simulink model "rtwdemo_advisor2"  (Simulink 6.0)
settings: Solver=FixedStepDiscrete  SolverMode=SingleTasking  StartTime=0.0  StopTime=4  FixedStep=1  RelTol=1e-3  AbsTol=1e-6
undefined symbols (not defined in the file or in its folder): DiscIntNeverNeededParam
libraries: simulink x4, rtwdemowidgets x1
settings Model: CovMetricSettings=d  Creator=The MathWorks Inc.  LastModifiedBy=batserve  ExtModeTrigMode=oneshot  ExtModeArmWhenConnect=off  ExtModeAutoUpdateStatusClock=off  ProdHWDeviceType=Specified
settings DataIOCC: LimitDataPoints=off  SaveOutput=off  SaveTime=off  SignalLoggingName=sigsOut
settings OptimizationCC: InlineParams=on  EnforceIntegerDowncast=off  ZeroExternalMemoryAtStartup=off  ZeroInternalMemoryAtStartup=off  OptimizeModelRefInitCode=on  LifeSpan=1
settings DebuggingCC: CheckExecutionContextPreStartOutputMsg=on  CheckExecutionContextRuntimeOutputMsg=on  SolverPrmCheckMsg=none  IntegerOverflowMsg=none  ParameterDowncastMsg=warning  ParameterOverflowMsg=warning  ParameterPrecisionLossMsg=none
settings HardwareCC: ProdBitPerInt=16  ProdHWDeviceType=Specified  TargetUnknown=on
settings RTWCC: SystemTargetFile=ert.tlc  GenCodeOnly=on  TemplateMakefile=ert_default_tmf  GenerateReport=on  RTWVerbose=off  ProcessScript=ert_make_rtw_hook  IncludeHyperlinkInReport=on  LaunchReport=on
settings CodeAppCC: IgnoreCustomStorageClasses=off  IncHierarchyInIds=on  IncDataTypeInIds=on
settings ERTTargetCC: TargetFcnLib=ansi_tfl_tmw.mat  GenFloatMathFcnCalls=ANSI_C  IncludeMdlTerminateFcn=off  SuppressErrorStatus=on  SupportContinuousTime=on  SupportNonInlinedSFcns=on  RootIOFormat=Individual Arguments  ERTCustomFileTemplate=example_file_process.tlc  InitialValueSource=Model

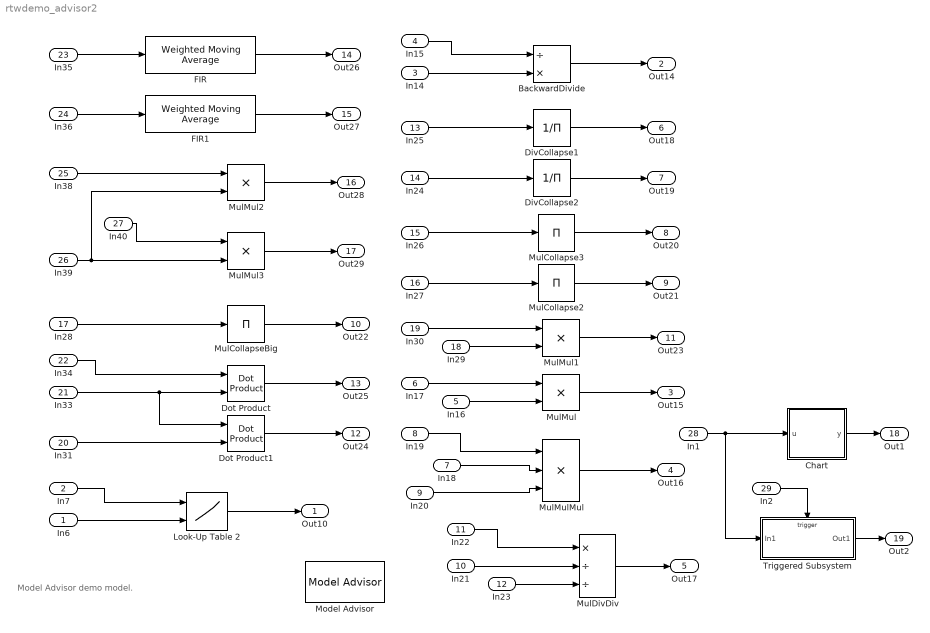
== system rtwdemo_advisor2 ==
  note: Model Advisor demo model.
  In6 : Inport  Port=1  PortDimensions=1  SampleTime=1  DataType=Specify via dialog  OutScaling=2^-10  LatchInput=off  Interpolate=off
  In7 : Inport  Port=2  PortDimensions=1  SampleTime=1  DataType=Specify via dialog  OutScaling=2^-10  LatchInput=off  Interpolate=off
  In14 : Inport  Port=3  PortDimensions=1  SampleTime=1  DataType=Specify via dialog  OutScaling=2^-10  LatchInput=off  Interpolate=off
  In15 : Inport  Port=4  PortDimensions=1  SampleTime=1  DataType=Specify via dialog  OutScaling=2^-10  LatchInput=off  Interpolate=off
  In16 : Inport  Port=5  PortDimensions=1  SampleTime=1  DataType=Specify via dialog  OutDataType=sfix(32)  OutScaling=2^-10  LatchInput=off  Interpolate=off
  In17 : Inport  Port=6  PortDimensions=1  SampleTime=1  DataType=Specify via dialog  OutScaling=2^-10  LatchInput=off  Interpolate=off
  In18 : Inport  Port=7  PortDimensions=1  SampleTime=1  DataType=Specify via dialog  OutScaling=2^-10  LatchInput=off  Interpolate=off
  In19 : Inport  Port=8  PortDimensions=1  SampleTime=1  DataType=Specify via dialog  OutScaling=2^-10  LatchInput=off  Interpolate=off
  In20 : Inport  Port=9  PortDimensions=1  SampleTime=1  DataType=Specify via dialog  OutScaling=2^-10  LatchInput=off  Interpolate=off
  In21 : Inport  Port=10  PortDimensions=1  SampleTime=1  DataType=Specify via dialog  OutScaling=2^-10  LatchInput=off  Interpolate=off
  In22 : Inport  Port=11  PortDimensions=1  SampleTime=1  DataType=Specify via dialog  OutScaling=2^-10  LatchInput=off  Interpolate=off
  In23 : Inport  Port=12  PortDimensions=1  SampleTime=1  DataType=Specify via dialog  OutScaling=2^-10  LatchInput=off  Interpolate=off
  In25 : Inport  Port=13  PortDimensions=1  SampleTime=1  DataType=Specify via dialog  OutScaling=2^-10  LatchInput=off  Interpolate=off
  In24 : Inport  Port=14  PortDimensions=2  SampleTime=1  DataType=Specify via dialog  OutScaling=2^-10  LatchInput=off  Interpolate=off
  In26 : Inport  Port=15  PortDimensions=3  SampleTime=1  DataType=Specify via dialog  OutScaling=2^-10  LatchInput=off  Interpolate=off
  In27 : Inport  Port=16  PortDimensions=2  SampleTime=1  DataType=Specify via dialog  OutScaling=2^-10  LatchInput=off  Interpolate=off
  In28 : Inport  Port=17  PortDimensions=2  SampleTime=1  DataType=Specify via dialog  OutDataType=sfix(32)  OutScaling=2^-10  LatchInput=off  Interpolate=off
  In29 : Inport  Port=18  PortDimensions=1  SampleTime=1  DataType=Specify via dialog  OutScaling=2^-10  LatchInput=off  Interpolate=off
  In30 : Inport  Port=19  PortDimensions=1  SampleTime=1  DataType=Specify via dialog  OutScaling=2^-10  LatchInput=off  Interpolate=off
  In31 : Inport  Port=20  PortDimensions=1  SampleTime=1  DataType=Specify via dialog  OutDataType=sfix(32)  OutScaling=2^-10  LatchInput=off  Interpolate=off
  In33 : Inport  Port=21  PortDimensions=1  SampleTime=1  DataType=Specify via dialog  OutScaling=2^-10  LatchInput=off  Interpolate=off
  In34 : Inport  Port=22  PortDimensions=1  SampleTime=1  DataType=Specify via dialog  OutScaling=2^-10  LatchInput=off  Interpolate=off
  In35 : Inport  Port=23  PortDimensions=1  SampleTime=1  DataType=Specify via dialog  OutDataType=sfix(32)  OutScaling=2^-10  LatchInput=off  Interpolate=off
  In36 : Inport  Port=24  PortDimensions=1  SampleTime=1  DataType=Specify via dialog  OutDataType=sfix(32)  OutScaling=2^-10  LatchInput=off  Interpolate=off
  In38 : Inport  Port=25  PortDimensions=1  SampleTime=1  DataType=Specify via dialog  OutScaling=1.01 * 2^-10  LatchInput=off  Interpolate=off
  In39 : Inport  Port=26  PortDimensions=1  SampleTime=1  DataType=Specify via dialog  OutScaling=2^-10  LatchInput=off  Interpolate=off
  In40 : Inport  Port=27  PortDimensions=1  SampleTime=1  DataType=Specify via dialog  OutScaling=[2^-10 1]  LatchInput=off  Interpolate=off
  In1 : Inport  Port=28  OutScaling=2^-10  LatchInput=off  Interpolate=off
  In2 : Inport  Port=29  DataType=boolean  OutScaling=2^-10  LatchInput=off  Interpolate=off
  BackwardDivide : Product  Inputs=/*  OutDataTypeMode=Specify via dialog  OutScaling=2^-10
  Chart : Stateflow chart  PropExecContextAcrossSSBoundary=on
  DivCollapse1 : Product  Inputs=/  OutDataTypeMode=Specify via dialog  OutScaling=2^-10
  DivCollapse2 : Product  Inputs=/  OutDataTypeMode=Specify via dialog  OutScaling=2^-10
  Dot Product : simulink/Math Operations/Dot Product  OutputDataTypeScalingMode=Specify via dialog  OutDataType=sfix(32)  OutScaling=2^-10  DoSatur=off
  Dot Product1 : simulink/Math Operations/Dot Product  OutputDataTypeScalingMode=Specify via dialog  OutDataType=sfix(32)  OutScaling=2^-10  DoSatur=off
  FIR : simulink/Discrete/Weighted Moving Average  mgainval=[0.1:0.1:1 0.9:-0.1:0.1]  vinit=0.0  samptime=-1  GainDataTypeScalingMode=Specify via dialog  GainDataType=sfix( 16 )  MatRadixGroup=Best Precision: Matrix-wise  GainScaling=2^-14  OutputDataTypeScalingMode=Specify via dialog  OutDataType=sfix(32)  OutScaling=2^-10  DoSatur=off
  FIR1 : simulink/Discrete/Weighted Moving Average  mgainval=[0.1:0.1:1 0.9:-0.1:0.1]  vinit=0.0  samptime=-1  GainDataTypeScalingMode=Specify via dialog  GainDataType=sfix( 16 )  MatRadixGroup=Best Precision: Matrix-wise  GainScaling=2^-14  OutputDataTypeScalingMode=Specify via dialog  OutDataType=sfix(32)  OutScaling=2^-20  DoSatur=off
  Look-Up Table 2 : Lookup2D  DialogController=Simulink.DDGSource  RowIndex=[1:3]  ColumnIndex=[1 2 7]  OutputValues=[4 5 6;16 19 20;10 18 23]  LookUpMeth=Interpolation-Use End Values  OutDataTypeMode=Specify via dialog  OutScaling=2^-10
  Model Advisor : rtwdemowidgets/Model Advisor  attrib_overrides={}
  MulCollapse2 : Product  Inputs=1  OutDataTypeMode=Specify via dialog  OutScaling=2^-10
  MulCollapse3 : Product  Inputs=*  OutDataTypeMode=Specify via dialog  OutScaling=2^-10
  MulCollapseBig : Product  Inputs=1  OutDataTypeMode=Specify via dialog  OutScaling=2^-10
  MulDivDiv : Product  Inputs=*//  OutDataTypeMode=Specify via dialog  OutScaling=2^-10
  MulMul : Product  OutDataTypeMode=Specify via dialog  OutScaling=2^-3
  MulMul1 : Product  OutDataTypeMode=Specify via dialog  OutScaling=2^-10
  MulMul2 : Product  OutDataTypeMode=Specify via dialog  OutScaling=2^-10
  MulMul3 : Product  OutDataTypeMode=Specify via dialog  OutScaling=2^-10
  MulMulMul : Product  Inputs=3  OutDataTypeMode=Specify via dialog  OutScaling=2^-10
  Triggered Subsystem : Subsystem  TreatAsAtomicUnit=on  PropExecContextAcrossSSBoundary=on
  Out10 : Outport
  Out14 : Outport  Port=2
  Out15 : Outport  Port=3
  Out16 : Outport  Port=4
  Out17 : Outport  Port=5
  Out18 : Outport  Port=6
  Out19 : Outport  Port=7
  Out20 : Outport  Port=8
  Out21 : Outport  Port=9
  Out22 : Outport  Port=10
  Out23 : Outport  Port=11
  Out24 : Outport  Port=12
  Out25 : Outport  Port=13
  Out26 : Outport  Port=14
  Out27 : Outport  Port=15
  Out28 : Outport  Port=16
  Out29 : Outport  Port=17
  Out1 : Outport  Port=18
  Out2 : Outport  Port=19
  wires:
  In6/1 -> Look-Up Table 2/2
  Look-Up Table 2/1 -> Out10/1
  In7/1 -> Look-Up Table 2/1
  In14/1 -> BackwardDivide/2
  BackwardDivide/1 -> Out14/1
  In15/1 -> BackwardDivide/1
  MulMul/1 -> Out15/1
  In17/1 -> MulMul/1
  In18/1 -> MulMulMul/2
  MulMulMul/1 -> Out16/1
  In19/1 -> MulMulMul/1
  In20/1 -> MulMulMul/3
  In21/1 -> MulDivDiv/2
  MulDivDiv/1 -> Out17/1
  In22/1 -> MulDivDiv/1
  In23/1 -> MulDivDiv/3
  DivCollapse1/1 -> Out18/1
  In25/1 -> DivCollapse1/1
  DivCollapse2/1 -> Out19/1
  In24/1 -> DivCollapse2/1
  MulCollapse3/1 -> Out20/1
  In26/1 -> MulCollapse3/1
  MulCollapse2/1 -> Out21/1
  In27/1 -> MulCollapse2/1
  MulCollapseBig/1 -> Out22/1
  In28/1 -> MulCollapseBig/1
  MulMul1/1 -> Out23/1
  In30/1 -> MulMul1/1
  In31/1 -> Dot Product1/2
  Dot Product1/1 -> Out24/1
  In33/1 -> Dot Product/2, Dot Product1/1
  Dot Product/1 -> Out25/1
  In34/1 -> Dot Product/1
  In35/1 -> FIR/1
  FIR/1 -> Out26/1
  In36/1 -> FIR1/1
  FIR1/1 -> Out27/1
  MulMul2/1 -> Out28/1
  In38/1 -> MulMul2/1
  In39/1 -> MulMul3/2, MulMul2/2
  MulMul3/1 -> Out29/1
  In40/1 -> MulMul3/1
  In16/1 -> MulMul/2
  In29/1 -> MulMul1/2
  In1/1 -> Chart/1(u), Triggered Subsystem/1(In1)
  Chart/1(y) -> Out1/1
  Triggered Subsystem/1(Out1) -> Out2/1
  In2/1 -> Triggered Subsystem/Trigger

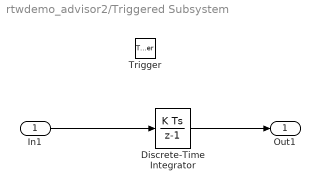
== system rtwdemo_advisor2/Triggered Subsystem ==
  In1 : Inport  Port=1  LatchInput=off
  Trigger : TriggerPort
  Discrete-Time Integrator : DiscreteIntegrator  SampleTime=-1  ICPrevOutput=DiscIntNeverNeededParam  ICPrevScaledInput=DiscIntNeverNeededParam
  Out1 : Outport
  wires:
  In1/1 -> Discrete-Time Integrator/1
  Discrete-Time Integrator/1 -> Out1/1

== stateflow chart Chart ==
  state B
  state A
  A -> B : {y=u*2;}
  (default) -> A
  data: u input int32 size=1; y output int32 size=1
